simulink model "armature_dcmotor"  (R2024b)
settings: Solver=VariableStepAuto  StartTime=0.0  StopTime=10.0  RelTol=1e-3
settings Model: Creator=Rj Avro Biswas  LastModifiedBy=Rj Avro Biswas

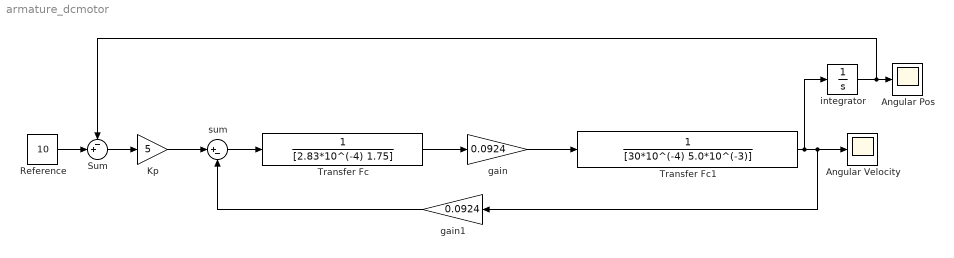
== system armature_dcmotor ==
  Angular Pos : Scope
  Angular Velocity : Scope
  Kp : Gain  Gain=5
  Reference : Constant  Value=10
  Sum : Sum  Inputs=-+|
  Transfer Fc : TransferFcn  Denominator=[2.83*10^(-4) 1.75]
  Transfer Fc1 : TransferFcn  Denominator=[30*10^(-4) 5.0*10^(-3)]
  gain : Gain  Gain=0.0924
  gain1 : Gain  Gain=0.0924
  integrator : Integrator
  sum : Sum  Inputs=|+-
  wires:
  Transfer Fc/1 -> gain/1
  gain/1 -> Transfer Fc1/1
  Transfer Fc1/1 -> integrator/1, gain1/1, Angular Velocity/1
  sum/1 -> Transfer Fc/1
  gain1/1 -> sum/2
  Reference/1 -> Sum/2
  integrator/1 -> Sum/1, Angular Pos/1
  Sum/1 -> Kp/1
  Kp/1 -> sum/1
